simulink model "field_simulator"  (R2020b)
settings: Solver=VariableStepAuto  StartTime=0.0  StopTime=T  RelTol=1e-3  AbsTol=1e-3  EnableMultiTasking=on
model workspace (MAT data in the model file):
  x10 = 0
undefined symbols (not defined in the file): X, Y, Z
libraries: vrlib x14, sm_lib x4, nesl_utility x2, visionsinks x1
settings Model: Creator=20204924  LastModifiedBy=20204924
settings SolverCC: AutoScaleAbsTol=off
settings DataIOCC: LimitDataPoints=on  MaxDataPoints=10000
settings OptimizationCC: LifeSpan=inf
settings DebuggingCC: AllowSymbolicDim=off  SFUnexpectedBacktrackingDiag=warning  SFNoUnconditionalDefaultTransitionDiag=warning  SFExecutionAtInitializationDiag=none  ArithmeticOperatorsInVariantConditions=warning
settings SFSimCC: SimUseLocalCustomCode=off  CustomCodeUndefinedFunction=UseInterfaceOnly
settings RTWCC: RTWUseLocalCustomCode=off
settings CodeAppCC: StateflowObjectComments=on
settings GRTTargetCC: TargetLangStandard=C89/C90 (ANSI)
settings ConfigComp: CovMetricSettings=dw  CovSaveCumulativeToWorkspaceVar=on  CovSaveSingleToWorkspaceVar=on  CovExternalEMLEnable=off  CovSFcnEnable=off
settings SimscapeCC: SimscapeLogType=all  SimscapeLogSimulationStatistics=on  SimscapeLogDataHistory=10000

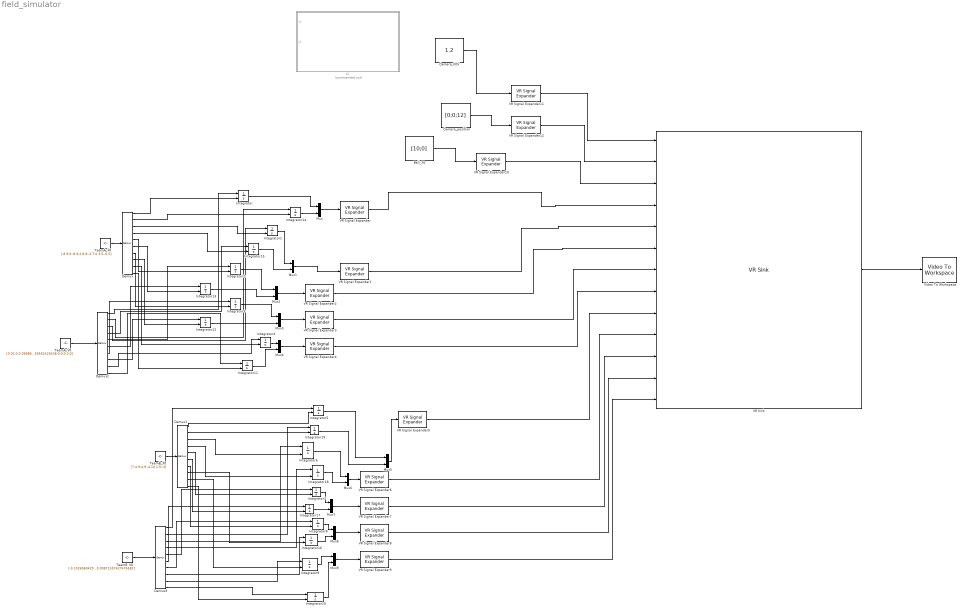
== system field_simulator ==
  A1 : Subsystem  Commented=on
  Ball_X0 : Constant  Value=[10;0]  VectorParams1D=off
  Camera_FOV : Constant  Value=1.2  VectorParams1D=off
  Camera_position : Constant  Value=[0;0;12]  VectorParams1D=off
  Demux{,1..3} (4 alike) : Demux  Outputs=10
  Integrator{,1..19} (20 alike) : Integrator  InitialConditionSource=external
  Mux{,1..9} (10 alike) : Mux  Inputs=2
  TeamA_V0 : Constant  Value=[0.02;0;0.0998629534754574;0.00523359562429438;0.0998629534754574;-0.00523359562429438;0;0;0.3;0]
  TeamA_X0 : Constant  Value=[-8.9;0;-8.9;2;8.8;-2;7;0.3;5;-0.5]
  TeamB_V0 : Constant  Value=[-0.102606042997701;-0.281907786235773;-0.00998629534754574;-0.000523359562429436;-0.0199725906950915;0.00104671912485888;-0.1;1.22464679914735e-17;-0.0996194698091746;0.00871557427476582]
  TeamB_X0 : Constant  Value=[7;4;9;4;9;-4;10;1;9;-3]
  VR Signal Expander{,1..10} (11 alike) : vrlib/VR Signal Expander  outwidth=3  outidx=[1 2]
  VR Signal Expander11 : vrlib/VR Signal Expander  outwidth=1  outidx=[1]
  VR Signal Expander12 : vrlib/VR Signal Expander  outwidth=3  outidx=[1 2 3]
  VR Sink : vrlib/VR Sink  InstantiateOnLoad=on  SampleTime=0.033  ViewEnable=on  RemoteChange=off  RemoteView=off  FieldsWritten=Custom_Top_Camera.fieldOfView.1.1.1.double#Custom_Top_Camera.position.3.1.1.double#Football2.translation.3.1.1.double#RedPlayer1.translation.3.1.1.double#RedPlayer2.translation.3.1.1.double#RedPlayer3.translation.3.1.1.double#RedPlayer4.translation.3.1.1.double#RedPlayer5.translation.3.1.1.double#YellowPlayer1.translation.3.1.1.double#YellowPlayer2.translation.3.1.1.double#YellowPlayer3.translation.3.1.1.double#YellowPlayer4.translation.3.1.1.double#YellowPlayer5.translation.3.1.1.double  WorldFileName=virtual_field.WRL  AutoView=off  VideoDimensions=[1080 1920]  AllowVariableSize=off  FigureProperties="{'Position', 'Name', 'Viewpoint', 'CameraBound', 'CameraDirection', 'CameraPosition', 'CameraUpVector', 'ZoomFactor', 'Antialiasing', 'Headlight', 'Lighting', 'NavPanel', 'Sound', 'StatusBar', 'Stereo3D', 'Stereo3DCameraOffset', 'Stereo3DHIT', 'ToolBar', 'Textures', 'Transparency', 'Triad', 'Wireframe', 'NavZones', 'NavMode', 'NavSpeed', 'CaptureFileFormat', 'CaptureFileName', 'Record2DCompressMethod', 'Record2DCompressQuality', 'Record2D', 'Record2DFileName', 'Record2DFPS'; [5.0000000000000000e+00   1.0539999999999986e+02   1.5360000000000000e+03   8.6400000000000000e+02], '', 'custom_top_view', 'on', [0.0000000000000000e+00   0.0000000000000000e+00  -1.0000000000000000e+00], [0.0000000000000000e+00   0.0000000000000000e+00   0.0000000000000000e+00], [0.0000000000000000e+00   1.0000000000000000e+00   0.0000000000000000e+00], [1.0000000000000000e+00], 'on', 'on', 'off', 'none', 'on', 'off', 'off', [1.0000000149011612e-01], [0.0000000000000000e+00], 'off', 'on', 'off', 'none', 'off', 'off', 'fly', 'normal', 'tif', '..\\images\\%f_anim_%n.png', 'auto', [7.5000000000000000e+01], 'off', '***video***', 'auto'}"
  Video To Workspace : visionsinks/Video To Workspace  VariableName=vout  NumInputs=1  DataLimit=2000  DecimationFactor=1  LogFi=off  InPortLabels=R|G|B
      settings: SourceProductBaseCode=VP
  wires:
  Mux/1 -> VR Signal Expander/1
  Demux/1 -> Integrator/2
  Demux/2 -> Integrator14/2
  Demux/3 -> Integrator1/2
  Mux1/1 -> VR Signal Expander1/1
  Demux/4 -> Integrator15/2
  Mux2/1 -> VR Signal Expander2/1
  Demux/5 -> Integrator2/2
  Demux/6 -> Integrator13/2
  Mux3/1 -> VR Signal Expander3/1
  Demux/7 -> Integrator3/2
  Demux/8 -> Integrator12/2
  Mux4/1 -> VR Signal Expander4/1
  Demux/9 -> Integrator4/2
  TeamA_X0/1 -> Demux/1
  Mux8/1 -> VR Signal Expander8/1
  Demux1/3 -> Integrator6/2
  Demux1/4 -> Integrator18/2
  Demux1/9 -> Integrator9/2
  Mux9/1 -> VR Signal Expander9/1
  Demux1/10 -> Integrator10/2
  Demux1/5 -> Integrator7/2
  Mux6/1 -> VR Signal Expander6/1
  Mux7/1 -> VR Signal Expander7/1
  Demux1/8 -> Integrator16/2
  Demux1/1 -> Integrator5/2
  Demux1/6 -> Integrator17/2
  Demux1/2 -> Integrator19/2
  TeamB_X0/1 -> Demux1/1
  Demux1/7 -> Integrator8/2
  Mux5/1 -> VR Signal Expander5/1
  Integrator/1 -> Mux/1
  Integrator1/1 -> Mux1/1
  Integrator2/1 -> Mux2/1
  Ball_X0/1 -> VR Signal Expander10/1
  Integrator3/1 -> Mux3/1
  Integrator4/1 -> Mux4/1
  Integrator5/1 -> Mux5/1
  Integrator6/1 -> Mux6/1
  Integrator7/1 -> Mux7/1
  Integrator8/1 -> Mux8/1
  Integrator9/1 -> Mux9/1
  Integrator10/1 -> Mux9/2
  Demux3/1 -> Integrator5/1
  Integrator11/1 -> Mux4/2
  Integrator12/1 -> Mux3/2
  Integrator13/1 -> Mux2/2
  Integrator14/1 -> Mux/2
  Integrator15/1 -> Mux1/2
  Integrator16/1 -> Mux8/2
  Integrator17/1 -> Mux7/2
  Integrator18/1 -> Mux6/2
  Integrator19/1 -> Mux5/2
  Demux/10 -> Integrator11/2
  TeamA_V0/1 -> Demux2/1
  Demux2/1 -> Integrator/1
  Demux2/2 -> Integrator14/1
  Demux2/3 -> Integrator1/1
  Demux2/4 -> Integrator15/1
  Demux2/5 -> Integrator2/1
  Demux2/6 -> Integrator13/1
  Demux2/7 -> Integrator3/1
  Demux2/8 -> Integrator12/1
  Demux2/9 -> Integrator4/1
  Demux2/10 -> Integrator11/1
  TeamB_V0/1 -> Demux3/1
  Demux3/2 -> Integrator19/1
  Demux3/3 -> Integrator6/1
  Demux3/4 -> Integrator18/1
  Demux3/5 -> Integrator7/1
  Demux3/6 -> Integrator17/1
  Demux3/10 -> Integrator10/1
  Demux3/9 -> Integrator9/1
  Demux3/8 -> Integrator16/1
  Demux3/7 -> Integrator8/1
  VR Signal Expander10/1 -> VR Sink/3
  VR Signal Expander/1 -> VR Sink/4
  VR Signal Expander1/1 -> VR Sink/5
  VR Signal Expander2/1 -> VR Sink/6
  VR Signal Expander3/1 -> VR Sink/7
  VR Signal Expander4/1 -> VR Sink/8
  VR Signal Expander5/1 -> VR Sink/9
  VR Signal Expander6/1 -> VR Sink/10
  VR Signal Expander7/1 -> VR Sink/11
  VR Signal Expander8/1 -> VR Sink/12
  VR Signal Expander9/1 -> VR Sink/13
  VR Signal Expander11/1 -> VR Sink/1
  VR Signal Expander12/1 -> VR Sink/2
  Camera_FOV/1 -> VR Signal Expander11/1
  Camera_position/1 -> VR Signal Expander12/1
  VR Sink/1 -> Video To Workspace/1

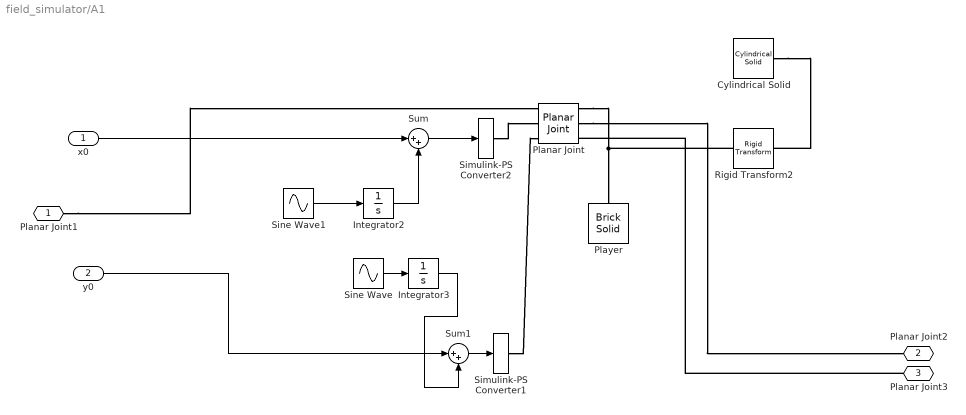
== system field_simulator/A1 ==
  x0 : Inport
  y0 : Inport  Port=2
  Cylindrical Solid : sm_lib/Body Elements/Cylindrical Solid  GraphicAmbientColor=[0.15 0.15 0.15 1.0]  BasedOnType=Density  CenterOfMass=[0 0 0]  CenterOfMassUnits=m  GraphicDiffuseColor=[0.7 0.2 0.5]  CylinderLength=0.01  CylinderLengthUnits=m  CylinderRadius=0.1  CylinderRadiusUnits=m  Density=1000  DensityUnits=kg/m^3  DoExposeReferenceFrame=on  GraphicEmissiveColor=[0.0 0.0 0.0 1.0]  ExportEntireGeometry=off  SerializedFrames=<Frames/>  MarkerShape=Sphere  MarkerSize=10  GraphicType=FromGeometry  InertiaType=CalculateFromGeometry  Mass=1  MassUnits=kg  MomentsOfInertia=[1 1 1]  MomentsOfInertiaUnits=kg*m^2  GraphicOpacity=1.0  ProductsOfInertia=[0 0 0]  ProductsOfInertiaUnits=kg*m^2  GraphicShininess=75  GraphicSpecularColor=[0.5 0.5 0.5 1.0]  GraphicVisPropType=SimpleVisualProperties
  Integrator2 : Integrator  InitialCondition=x10
  Integrator3 : Integrator
  Planar Joint : sm_lib/Joints/Planar Joint  JointMode=Normal  SenseConstraintForce=off  SenseConstraintForceX=off  SenseConstraintForceY=off  SenseConstraintForceZ=off  SenseConstraintTorque=off  SenseConstraintTorqueX=off  SenseConstraintTorqueY=off  SenseConstraintTorqueZ=off  SenseTotalForce=off  SenseTotalForceX=off  SenseTotalForceY=off  SenseTotalForceZ=off  SenseTotalTorque=off  SenseTotalTorqueX=off  SenseTotalTorqueY=off  SenseTotalTorqueZ=off  CompositeWrenchDir=FollowerOnBase  CompositeWrenchFrame=BaseFrame  PxEquilibriumPosition=0  PxEquilibriumPositionUnits=m  PxSpringStiffness=0  PxSpringStiffnessUnits=N/m  PxDampingCoefficient=0  PxDampingCoefficientUnits=N/(m/s)  PxTorqueActuationMode=ComputedTorque  PxMotionActuationMode=InputMotion  PxSensePosition=on  PxSenseVelocity=off  PxSenseAcceleration=off  PxSenseTorqueForce=off  PxSenseLowerLimitTorqueForce=off  PxSenseUpperLimitTorqueForce=off  PxLowerLimitSpecify=off  PxLowerLimitBound=-1  PxLowerLimitBoundUnits=m  PxLowerLimitStiffness=1e6  PxLowerLimitStiffnessUnits=N/m  PxLowerLimitDamping=1e3  PxLowerLimitDampingUnits=N/(m/s)  PxLowerLimitTransitionRegionWidth=1e-4  PxLowerLimitTransitionRegionWidthUnits=m  PxUpperLimitSpecify=off  PxUpperLimitBound=1  PxUpperLimitBoundUnits=m  PxUpperLimitStiffness=1e6  PxUpperLimitStiffnessUnits=N/m  PxUpperLimitDamping=1e3  PxUpperLimitDampingUnits=N/(m/s)  PxUpperLimitTransitionRegionWidth=1e-4  PxUpperLimitTransitionRegionWidthUnits=m  PxPositionTargetSpecify=on  PxPositionTargetPriority=Low  PxPositionTargetValue=1  PxPositionTargetValueUnits=m  PxVelocityTargetSpecify=off  PxVelocityTargetPriority=High  PxVelocityTargetValue=0  PxVelocityTargetValueUnits=m/s  PyEquilibriumPosition=0  PyEquilibriumPositionUnits=m  PySpringStiffness=0  PySpringStiffnessUnits=N/m  PyDampingCoefficient=0  PyDampingCoefficientUnits=N/(m/s)  PyTorqueActuationMode=ComputedTorque  PyMotionActuationMode=InputMotion  PySensePosition=on  PySenseVelocity=off  PySenseAcceleration=off  PySenseTorqueForce=off  PySenseLowerLimitTorqueForce=off  PySenseUpperLimitTorqueForce=off  PyLowerLimitSpecify=off  PyLowerLimitBound=-1  PyLowerLimitBoundUnits=m  PyLowerLimitStiffness=1e6  PyLowerLimitStiffnessUnits=N/m  PyLowerLimitDamping=1e3  PyLowerLimitDampingUnits=N/(m/s)  PyLowerLimitTransitionRegionWidth=1e-4  PyLowerLimitTransitionRegionWidthUnits=m  PyUpperLimitSpecify=off  PyUpperLimitBound=1  PyUpperLimitBoundUnits=m  PyUpperLimitStiffness=1e6  PyUpperLimitStiffnessUnits=N/m  PyUpperLimitDamping=1e3  PyUpperLimitDampingUnits=N/(m/s)  PyUpperLimitTransitionRegionWidth=1e-4  PyUpperLimitTransitionRegionWidthUnits=m  PyPositionTargetSpecify=on  PyPositionTargetPriority=Low  PyPositionTargetValue=-1  PyPositionTargetValueUnits=m  PyVelocityTargetSpecify=off  PyVelocityTargetPriority=High  PyVelocityTargetValue=0  PyVelocityTargetValueUnits=m/s  RzEquilibriumPosition=0  RzEquilibriumPositionUnits=deg  RzSpringStiffness=0  RzSpringStiffnessUnits=N*m/deg  RzDampingCoefficient=0  RzDampingCoefficientUnits=N*m/(deg/s)  RzTorqueActuationMode=NoTorque  RzMotionActuationMode=ComputedMotion  RzSensePosition=off  RzSenseVelocity=off  RzSenseAcceleration=off  RzSenseTorqueForce=off  RzSenseLowerLimitTorqueForce=off  RzSenseUpperLimitTorqueForce=off  RzLowerLimitSpecify=off  RzLowerLimitBound=-90  RzLowerLimitBoundUnits=deg  RzLowerLimitStiffness=1e4  RzLowerLimitStiffnessUnits=N*m/deg  RzLowerLimitDamping=10  RzLowerLimitDampingUnits=N*m/(deg/s)  RzLowerLimitTransitionRegionWidth=0.1  RzLowerLimitTransitionRegionWidthUnits=deg  RzUpperLimitSpecify=off  RzUpperLimitBound=90  RzUpperLimitBoundUnits=deg  RzUpperLimitStiffness=1e4  RzUpperLimitStiffnessUnits=N*m/deg  RzUpperLimitDamping=10  RzUpperLimitDampingUnits=N*m/(deg/s)  RzUpperLimitTransitionRegionWidth=0.1  RzUpperLimitTransitionRegionWidthUnits=deg  RzPositionTargetSpecify=off  RzPositionTargetPriority=High  RzPositionTargetValue=0  RzPositionTargetValueUnits=deg  RzVelocityTargetSpecify=off  RzVelocityTargetPriority=High  RzVelocityTargetValue=0  RzVelocityTargetValueUnits=deg/s
  Player : sm_lib/Body Elements/Brick Solid  GraphicAmbientColor=[0.15 0.15 0.15 1.0]  BasedOnType=Density  BrickDimensions=[0.5 0.5 0.8]  BrickDimensionUnits=m  CenterOfMass=[0 0 0]  CenterOfMassUnits=m  GraphicDiffuseColor=[0.2 0.2 0.2]  Density=1000  DensityUnits=kg/m^3  DoExposeReferenceFrame=on  GraphicEmissiveColor=[0.0 0.0 0.0 1.0]  ExportEntireGeometry=off  SerializedFrames=<Frames/>  MarkerShape=Sphere  MarkerSize=10  GraphicType=FromGeometry  InertiaType=CalculateFromGeometry  Mass=1  MassUnits=kg  MomentsOfInertia=[1 1 1]  MomentsOfInertiaUnits=kg*m^2  GraphicOpacity=1.0  ProductsOfInertia=[0 0 0]  ProductsOfInertiaUnits=kg*m^2  GraphicShininess=75  GraphicSpecularColor=[0.5 0.5 0.5 1.0]  GraphicVisPropType=SimpleVisualProperties
  Rigid Transform2 : sm_lib/Frames and Transforms/Rigid Transform  TranslationMethod=Cartesian  TranslationStandardOffset=0  TranslationLengthUnit=m  TranslationStandardAxis=+Z  TranslationCartesianOffset=[0 0 0.4]  TranslationROffset=0  TranslationROffsetUnits=m  TranslationZOffset=0  TranslationZOffsetUnits=m  TranslationThetaOffset=0  TranslationThetaOffsetUnits=deg  RotationMethod=None  RotationAngleUnits=deg  RotationStandardAxis=+Z  RotationAngle=0.0  RotationArbitraryAxis=[0 0 1]  FollAlignAxisA=+X  BaseAlignAxisA=+Y  FollAlignAxisB=+Y  BaseAlignAxisB=+Z  RotationSequenceAxes=FollowerAxes  RotationSequence=XYX  RotationSequenceAngles=[0 0 0]  RotationSequenceAnglesUnits=deg  RotationMatrix=[1 0 0; 0 1 0; 0 0 1]
  Simulink-PS Converter1 : nesl_utility/Simulink-PS Converter  PhysicalDomain=network_engine_domain  SubClassName=ps_input  LeftPortType=input  RightPortType=output  PseudoPeriodic=off  Frequencies=[]  NoiseDistribution=none  NoiseParameters=[]  Unit=1  AffineConversion=off  FilteringAndDerivatives=filter  SimscapeFilterOrder=2  InputFilterTimeConstant=0.001  UdotUserProvided=1
  Simulink-PS Converter2 : nesl_utility/Simulink-PS Converter  PhysicalDomain=network_engine_domain  SubClassName=ps_input  LeftPortType=input  RightPortType=output  PseudoPeriodic=off  Frequencies=[]  NoiseDistribution=none  NoiseParameters=[]  Unit=1  AffineConversion=off  FilteringAndDerivatives=filter  SimscapeFilterOrder=2  InputFilterTimeConstant=0.001  UdotUserProvided=1
  Sine Wave : Sin  Amplitude=0.01  Frequency=0.1  Phase=1.57  SampleTime=0
  Sine Wave1 : Sin  Amplitude=0.5  Frequency=0.1  SampleTime=0
  Sum : Sum  Inputs=|++
  Sum1 : Sum  Inputs=|++
  Planar Joint1 : PMIOPort  Side=Left
  Planar Joint2 : PMIOPort  Port=2  Side=Right
  Planar Joint3 : PMIOPort  Port=3  Side=Right
  wires:
  Integrator2/1 -> Sum/2
  Sine Wave/1 -> Integrator3/1
  Sum/1 -> Simulink-PS Converter2/1
  Sine Wave1/1 -> Integrator2/1
  Integrator3/1 -> Sum1/2
  Sum1/1 -> Simulink-PS Converter1/1
  x0/1 -> Sum/1
  y0/1 -> Sum1/1
  connections:
  Cylindrical Solid/RConn1 -- Rigid Transform2/RConn1
  Simulink-PS Converter2/RConn1 -- Planar Joint/LConn2
  Planar Joint/RConn1 -- Player/RConn1 -- Rigid Transform2/LConn1
  Simulink-PS Converter1/RConn1 -- Planar Joint/LConn3
  Planar Joint1/RConn1 -- Planar Joint/LConn1
  Planar Joint/RConn2 -- Planar Joint2/RConn1
  Planar Joint3/RConn1 -- Planar Joint/RConn3
